simulink model "task4_lab13"  (R2021a)
settings: Solver=VariableStepAuto  StartTime=0.0  StopTime=10.0  RelTol=1e-3
settings Model: Creator=reemb  LastModifiedBy=reemb

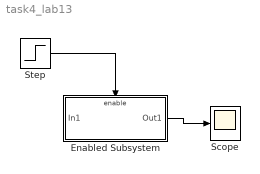
== system task4_lab13 ==
  Enabled Subsystem : Subsystem  TreatAsAtomicUnit=on
  Scope : Scope
  Step : Step  Time=5  SampleTime=0
  wires:
  Step/1 -> Enabled Subsystem/Enable
  Enabled Subsystem/1(Out1) -> Scope/1

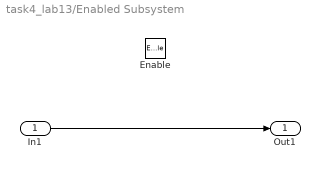
== system task4_lab13/Enabled Subsystem ==
  In1 : Inport
  Enable : EnablePort
  Out1 : Outport  InitialOutput=10
  wires:
  In1/1 -> Out1/1
